simulink model "Microgrid_LCTLM_server"  (R2025b)
settings: Solver=ode3  StartTime=0.0  StopTime=1  FixedStep=params.sampleTime  RelTol=1e-3
InitFcn:
  | unitlmModelFile = get_param(bdroot, 'FileName');
  | if ~isempty(unitlmModelFile), addpath(fileparts(unitlmModelFile)); end
  | initialise_optimised_tlm_interface();
  | clear unitlmModelFile
StartFcn:
  | unitlmModelFile = get_param(bdroot, 'FileName'); if ~isempty(unitlmModelFile), addpath(fileparts(unitlmModelFile)); end; try, if exist('unitlm_timing_probe', 'file') == 2, unitlm_timing_probe('start', 'server', bdroot); else, warning('uniTLM:TimingProbeNotFound', 'unitlm_timing_probe.m not found on MATLAB path; timing probe disabled.'); end; catch unitlmTimingError, warning('uniTLM:TimingProbeFailed', 'unitlm_timing_probe failed: %s', unitlmTimingError.message); end; clear unitlmModelFile
StopFcn:
  | unitlmModelFile = get_param(bdroot, 'FileName'); if ~isempty(unitlmModelFile), addpath(fileparts(unitlmModelFile)); end; try, if exist('unitlm_timing_probe', 'file') == 2, unitlm_timing_probe('stop', 'server', bdroot); else, warning('uniTLM:TimingProbeNotFound', 'unitlm_timing_probe.m not found on MATLAB path; timing probe disabled.'); end; catch unitlmTimingError, warning('uniTLM:TimingProbeFailed', 'unitlm_timing_probe failed: %s', unitlmTimingError.message); end; clear unitlmModelFile
  | %% StopFcn: save TLM server-side results
  | 
  | modelName = bdroot;
  | modelFile = get_param(modelName, 'FileName');
  | 
  | if isempty(modelFile)
  |     modelDir = pwd;
  | else
  |     modelDir = fileparts(modelFile);
  | end
  | 
  | resultDir = fullfile(modelDir, 'result');
  | 
  | if ~exist(resultDir, 'dir')
  |     mkdir(resultDir);
  | end
  | 
  | % Server-side workspace variables
  | variableNames = {
  |     'server_voltage'
  |     'server_current'
  |     'server_PQ'
  | };
  | 
  | serverTLMData = struct();
  | 
  | for k = 1:numel(variableNames)
  | 
  |     originalName = variableNames{k};
  |     saveName = [originalName, '_TLM'];
  | 
  |     if evalin('base', sprintf('exist(''%s'', ''var'')', originalName))
  |         serverTLMData.(saveName) = evalin('base', originalName);
  |     else
  |         warning( ...
  |             'StopFcn:MissingVariable', ...
  |             'Variable "%s" was not found in the base workspace.', ...
  |             originalName);
  |     end
  | end
  | 
  | % Save to result/server_TLM.mat
  | saveFile = fullfile(resultDir, 'server_TLM.mat');
  | save(saveFile, '-struct', 'serverTLMData');
  | 
  | fprintf('TLM server-side results saved to:\n%s\n', saveFile);
values from neighbouring files (symbols this model uses):
  Cf = Cf_pu*Cb    [initialize_unitlm_microgrid.m]
  f = logspace(log10(fMin), log10(fMax), nFrequency).'    [fit_non_heaviside_line_rational.m]    (also in initialize_unitlm_microgrid.m = 50)
  fsw1 = 10e3    (= 10000)    [initialize_unitlm_microgrid.m]
  hr_lp_a = interface.hr_lp_a    [initialise_optimised_tlm_interface.m]
  hr_lp_b = interface.hr_lp_b    [initialise_optimised_tlm_interface.m]
  Ip = 2*P/(3*Vp)    [initialize_unitlm_microgrid.m]
  L1 = L1_pu*Lb    [initialize_unitlm_microgrid.m]
  L2 = L2_pu*Lb    [initialize_unitlm_microgrid.m]
  L3 = L3_pu*Lb    [initialize_unitlm_microgrid.m]
  L4 = L4_pu*Lb    [initialize_unitlm_microgrid.m]
  L_leakageinductance_1 = windingInductance(primaryWindingIndex)    [initialise_optimised_tlm_interface.m]
  L_magnetisation_1 = transformer.LmPu*primaryZbase/omegaNominal    [initialise_optimised_tlm_interface.m]
  L_remain_server = interface.L_remain_server    [initialise_optimised_tlm_interface.m]
  Lc = Lc_pu*Lb    [initialize_unitlm_microgrid.m]
  Lf2 = Lf2_pu*Lb    [initialize_unitlm_microgrid.m]
  line_aHr = interface.line_aHr    [initialise_optimised_tlm_interface.m]    (also in initialize_unitlm_microgrid.m = real(line_aHr))
  line_aZc = interface.line_aZc    [initialise_optimised_tlm_interface.m]    (also in initialize_unitlm_microgrid.m = real(line_aZc))
  line_bHr = interface.line_bHr    [initialise_optimised_tlm_interface.m]    (also in initialize_unitlm_microgrid.m = real(line_bHr))
  line_bZc = interface.line_bZc    [initialise_optimised_tlm_interface.m]    (also in initialize_unitlm_microgrid.m = real(line_bZc))
  P = 5e6    (= 5000000)    [initialize_unitlm_microgrid.m]
  params = varargin{1}    [Client_co.m]    (also in Client_co_TLM.m; Server_co.m; Server_co_TLM.m; initialise_optimised_tlm_interface.m = config.cosimParams)
  R1 = R1_pu*Zb    [initialize_unitlm_microgrid.m]
  R2 = R2_pu*Zb    [initialize_unitlm_microgrid.m]
  R3 = R3_pu*Zb    [initialize_unitlm_microgrid.m]
  R4 = R4_pu*Zb    [initialize_unitlm_microgrid.m]
  R_copperloss_1 = windingResistance(primaryWindingIndex)    [initialise_optimised_tlm_interface.m]
  R_coreloss_1 = transformer.RmPu*primaryZbase    [initialise_optimised_tlm_interface.m]
  R_remain_server = interface.R_remain_server    [initialise_optimised_tlm_interface.m]
  Rbreaker = Rbreaker_pu*Zb    [initialize_unitlm_microgrid.m]
  Rdamp = Rf    [initialize_unitlm_microgrid.m]
  Rf = Rf_pu*Zb    [initialize_unitlm_microgrid.m]
  Rload1 = Vp/Ip    [initialize_unitlm_microgrid.m]
  Rload2 = Vp/Ip    [initialize_unitlm_microgrid.m]
  Rload3 = Vp/Ip    [initialize_unitlm_microgrid.m]
  Rv_pu = 0.1    [initialize_unitlm_microgrid.m]
  Sxfmr = 6.3e6    (= 6300000)    [initialize_unitlm_microgrid.m]
  Vac = sqrt(2)*Vline/sqrt(3)    [initialize_unitlm_microgrid.m]
  Vhv = 66e3    (= 66000)    [initialize_unitlm_microgrid.m]
  Vline = 690    [initialize_unitlm_microgrid.m]
  Vp = Vac    [initialize_unitlm_microgrid.m]
  Wb = 2*pi*f    (= 314.159265359)    [initialize_unitlm_microgrid.m]
  Xv_pu = 0.3    [initialize_unitlm_microgrid.m]
  Zc_base_L = interface.Zc_base_L    [initialise_optimised_tlm_interface.m]
  Zc_base_R = interface.Zc_base_R    [initialise_optimised_tlm_interface.m]
undefined symbols (not defined in the file or in its folder): DiscIntNeverNeededParam, DPL, dspblkCoreblockFVToolHelper, gcbh, Lline1
libraries: spsThreePhaseSeriesRLCBranchLib x18, spsControlledVoltageSourceLib x12, spsThreePhaseVIMeasurementLib x7, spsabctodq0Lib x6, simulink x4, slpidlib x4, spsThreePhaseBreakerLib x4, SimplusGT x3, spsThreePhaseTransformerTwoWindingsLib x3, spsPower3phInstantaneousLib x2, spsdq0toabcLib x2, spsDistributedParametersLineLib x1
(part 2 of 4)

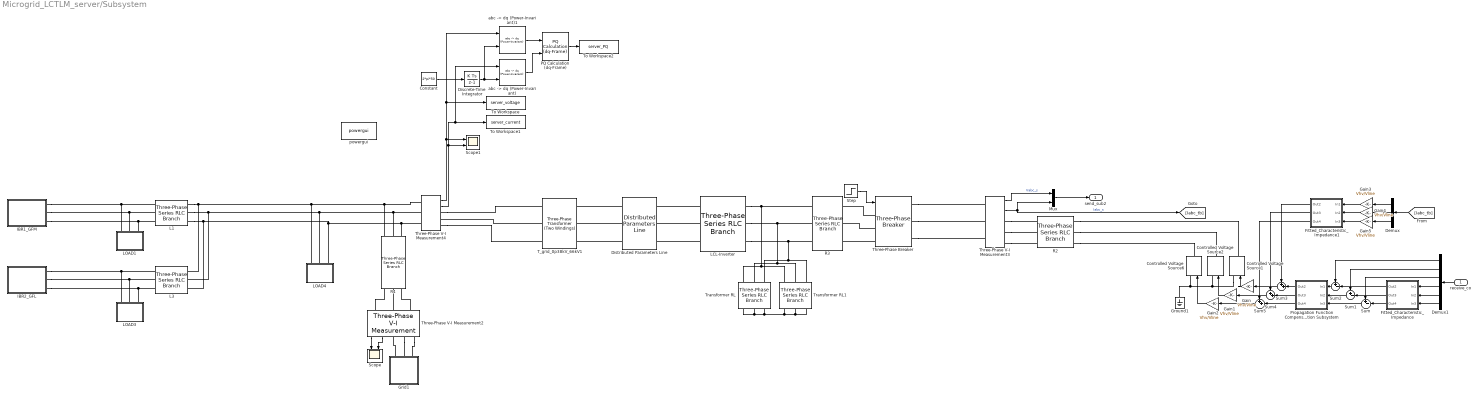
== system Microgrid_LCTLM_server/Subsystem ==
  receive_co : Inport
  Constant : Constant  Value=2*pi*50
  Controlled Voltage Source1 : spsControlledVoltageSourceLib/Controlled Voltage Source  Initialize=on  Source_Type=AC  Amplitude=0  Phase=0  Frequency=0  Measurements=None
  Controlled Voltage Source2 : spsControlledVoltageSourceLib/Controlled Voltage Source  Initialize=on  Source_Type=AC  Amplitude=0  Phase=0  Frequency=0  Measurements=None
  Controlled Voltage Source6 : spsControlledVoltageSourceLib/Controlled Voltage Source  Initialize=on  Source_Type=AC  Amplitude=0  Phase=0  Frequency=0  Measurements=None
  Demux : Demux  Outputs=3
  Demux1 : Demux  Outputs=6
  Discrete-Time Integrator : DiscreteIntegrator  SampleTime=-1  ICPrevOutput=DiscIntNeverNeededParam  ICPrevScaledInput=DiscIntNeverNeededParam
  Distributed Parameters Line : spsDistributedParametersLineLib/Distributed Parameters Line  Phases=3  Length=DPL.originalLength  Frequency=DPL.freq  Resistance=DPL.R  Inductance=DPL.L  Capacitance=DPL.C  x1=[-0.0002325 0 0 0;-0.000232 0 0 0;-0.0002315 0 0 0;-0.000231 0 0 0;-0.0002305 0 0 0;-0.00023 0 0 0;-0.0002295 0 0 0;-0.000229 0 0 0;-0.0002285 0 0 0;-0.000228 0 0 0;-0.0002275 0 0 0;-0.000227 0 0 0;-0.0002265 0 0 0;-0.000226 0 0 0;-0.0002255 0 0 0;-0.000225 0 0 0;-0.0002245 0 0 0;-0.000224 0 0 0;-0.0002235 0 0 0;-0.000223 0 0 0;-0.0002225 0 0 0;-0.000222 0 0 0;-0.0002215 0 0 0;-0.000221 0 0 0;-0.0002205 0 0 0;-0.00022 0 0 0;-0.0002195 0 0 0;-0.000219 0 0 0;-0.0002185 0 0 0;-0.000218 0 0 0;-0.0002175 0 0 0;-0.000217 0 0 0;-0.0002165 0 0 0;-0.000216 0 0 0;-0.0002155 0 0 0;-0.000215 0 0 0;-0.0002145 0 0 0;-0.000214 0 0 0;-0.0002135 0 0 0;-0.000213 0 0 0;-0.0002125 0 0 0;-0.000212 0 0 0;-0.0002115 0 0 0;-0.000211 0 0 0;-0.0002105 0 0 0;-0.00021 0 0 0;-0.0002095 0 0 0;-0.000209 0 0 0;-0.0002085 0 0 0;-0.000208 0 0 0;-0.0002075 0 0 0;-0.000207 0 0 0;-0.0002065 0 0 0;-0.000206 0 0 0;-0.0002055 0 0 0;-0.000205 0 0 0;-0.0002045 0 0 0;-0.000204 0 0 0;-0.0002035 0 0 0;-0.000203 0 0 0;-0.0002025 0 0 0;-0.000202 0 0 0;-0.0002015 0 0 0;-0.000201 0 0 0;-0.0002005 0 0 0;-0.0002 0 0 0;-0.0001995 0 0 0;-0.000199 0 0 0;-0.0001985 0 0 0;-0.000198 0 0 0;-0.0001975 0 0 0;-0.000197 0 0 0;-0.0001965 0 0 0;-0.000196 0 0 0;-0.0001955 0 0 0;-0.000195 0 0 0;-0.0001945 0 0 0;-0.000194 0 0 0;-0.0001935 0 0 0;-0.000193 0 0 0;-0.0001925 0 0 0;-0.000192 0 0 0;-0.0001915 0 0 0;-0.000191 0 0 0;-0.0001905 0 0 0;-0.00019 0 0 0;-0.0001895 0 0 0;-0.000189 0 0 0;-0.0001885 0 0 0;-0.000188 0 0 0;-0.0001875 0 0 0;-0.000187 0 0 0;-0.0001865 0 0 0;-0.000186 0 0 0;-0.0001855 0 0 0;-0.000185 0 0 0;-0.0001845 0 0 0;-0.000184 0 0 0;-0.0001835 0 0 0;-0.000183 0 0 0;-0.0001825 0 0 0;-0.000182 0 0 0;-0.0001815 0 0 0;-0.000181 0 0 0;-0.0001805 0 0 0;-0.00018 0 0 0;-0.0001795 0 0 0;-0.000179 0 0 0;-0.0001785 0 0 0;-0.000178 0 0 0;-0.0001775 0 0 0;-0.000177 0 0 0;-0.0001765 0 0 0;-0.000176 0 0 0;-0.0001755 0 0 0;-0.000175 0 0 0;-0.0001745 0 0 0;-0.000174 0 0 0;-0.0001735 0 0 0;-0.000173 0 0 0;-0.0001725 0 0 0;-0.000172 0 0 0;-0.0001715 0 0 0;-0.000171 0 0 0;-0.0001705 0 0 0;-0.00017 0 0 0;-0.0001695 0 0 0;-0.000169 0 0 0;-0.0001685 0 0 0;-0.000168 0 0 0;-0.0001675 0 0 0;-0.000167 0 0 0;-0.0001665 0 0 0;-0.000166 0 0 0;-0.0001655 0 0 0;-0.000165 0 0 0;-0.0001645 0 0 0;-0.000164 0 0 0;-0.0001635 0 0 0;-0.000163 0 0 0;-0.0001625 0 0 0;-0.000162 0 0 0;-0.0001615 0 0 0;-0.000161 0 0 0;-0.0001605 0 0 0;-0.00016 0 0 0;-0.0001595 0 0 0;-0.000159 0 0 0;-0.0001585 0 0 0;-0.000158 0 0 0;-0.0001575 0 0 0;-0.000157 0 0 0;-0.0001565 0 0 0;-0.000156 0 0 0;-0.0001555 0 0 0;-0.000155 0 0 0;-0.0001545 0 0 0;-0.000154 0 0 0;-0.0001535 0 0 0;-0.000153 0 0 0;-0.0001525 0 0 0;-0.000152 0 0 0;-0.0001515 0 0 0;-0.000151 0 0 0;-0.0001505 0 0 0;-0.00015 0 0 0;-0.0001495 0 0 0;-0.000149 0 0 0;-0.0001485 0 0 0;-0.000148 0 0 0;-0.0001475 0 0 0;-0.000147 0 0 0;-0.0001465 0 0 0;-0.000146 0 0 0;-0.0001455 0 0 0;-0.000145 0 0 0;-0.0001445 0 0 0;-0.000144 0 0 0;-0.0001435 0 0 0;-0.000143 0 0 0;-0.0001425 0 0 0;-0.000142 0 0 0;-0.0001415 0 0 0;-0.000141 0 0 0;-0.0001405 0 0 0;-0.00014 0 0 0;-0.0001395 0 0 0;-0.000139 0 0 0;-0.0001385 0 0 0;-0.000138 0 0 0;-0.0001375 0 0 0;-0.000137 0 0 0;-0.0001365 0 0 0;-0.000136 0 0 0;-0.0001355 0 0 0;-0.000135 0 0 0;-0.0001345 0 0 0;-0.000134 0 0 0;-0.0001335 0 0 0;-0.000133 0 0 0;-0.0001325 0 0 0;-0.000132 0 0 0;-0.0001315 0 0 0;-0.000131 0 0 0;-0.0001305 0 0 0;-0.00013 0 0 0;-0.0001295 0 0 0;-0.000129 0 0 0;-0.0001285 0 0 0;-0.000128 0 0 0;-0.0001275 0 0 0;-0.000127 0 0 0;-0.0001265 0 0 0;-0.000126 0 0 0;-0.0001255 0 0 0;-0.000125 0 0 0;-0.0001245 0 0 0;-0.000124 0 0 0;-0.0001235 0 0 0;-0.000123 0 0 0;-0.0001225 0 0 0;-0.000122 0 0 0;-0.0001215 0 0 0;-0.000121 0 0 0;-0.0001205 0 0 0;-0.00012 0 0 0;-0.0001195 0 0 0;-0.000119 0 0 0;-0.0001185 0 0 0;-0.000118 0 0 0;-0.0001175 0 0 0;-0.000117 0 0 0;-0.0001165 0 0 0;-0.000116 0 0 0;-0.0001155 0 0 0;-0.000115 0 0 0;-0.0001145 0 0 0;-0.000114 0 0 0;-0.0001135 0 0 0;-0.000113 0 0 0;-0.0001125 0 0 0;-0.000112 0 0 0;-0.0001115 0 0 0 ...(+3413 chars)]  x2=[-0.0002325 0 0 0;-0.000232 0 0 0;-0.0002315 0 0 0;-0.000231 0 0 0;-0.0002305 0 0 0;-0.00023 0 0 0;-0.0002295 0 0 0;-0.000229 0 0 0;-0.0002285 0 0 0;-0.000228 0 0 0;-0.0002275 0 0 0;-0.000227 0 0 0;-0.0002265 0 0 0;-0.000226 0 0 0;-0.0002255 0 0 0;-0.000225 0 0 0;-0.0002245 0 0 0;-0.000224 0 0 0;-0.0002235 0 0 0;-0.000223 0 0 0;-0.0002225 0 0 0;-0.000222 0 0 0;-0.0002215 0 0 0;-0.000221 0 0 0;-0.0002205 0 0 0;-0.00022 0 0 0;-0.0002195 0 0 0;-0.000219 0 0 0;-0.0002185 0 0 0;-0.000218 0 0 0;-0.0002175 0 0 0;-0.000217 0 0 0;-0.0002165 0 0 0;-0.000216 0 0 0;-0.0002155 0 0 0;-0.000215 0 0 0;-0.0002145 0 0 0;-0.000214 0 0 0;-0.0002135 0 0 0;-0.000213 0 0 0;-0.0002125 0 0 0;-0.000212 0 0 0;-0.0002115 0 0 0;-0.000211 0 0 0;-0.0002105 0 0 0;-0.00021 0 0 0;-0.0002095 0 0 0;-0.000209 0 0 0;-0.0002085 0 0 0;-0.000208 0 0 0;-0.0002075 0 0 0;-0.000207 0 0 0;-0.0002065 0 0 0;-0.000206 0 0 0;-0.0002055 0 0 0;-0.000205 0 0 0;-0.0002045 0 0 0;-0.000204 0 0 0;-0.0002035 0 0 0;-0.000203 0 0 0;-0.0002025 0 0 0;-0.000202 0 0 0;-0.0002015 0 0 0;-0.000201 0 0 0;-0.0002005 0 0 0;-0.0002 0 0 0;-0.0001995 0 0 0;-0.000199 0 0 0;-0.0001985 0 0 0;-0.000198 0 0 0;-0.0001975 0 0 0;-0.000197 0 0 0;-0.0001965 0 0 0;-0.000196 0 0 0;-0.0001955 0 0 0;-0.000195 0 0 0;-0.0001945 0 0 0;-0.000194 0 0 0;-0.0001935 0 0 0;-0.000193 0 0 0;-0.0001925 0 0 0;-0.000192 0 0 0;-0.0001915 0 0 0;-0.000191 0 0 0;-0.0001905 0 0 0;-0.00019 0 0 0;-0.0001895 0 0 0;-0.000189 0 0 0;-0.0001885 0 0 0;-0.000188 0 0 0;-0.0001875 0 0 0;-0.000187 0 0 0;-0.0001865 0 0 0;-0.000186 0 0 0;-0.0001855 0 0 0;-0.000185 0 0 0;-0.0001845 0 0 0;-0.000184 0 0 0;-0.0001835 0 0 0;-0.000183 0 0 0;-0.0001825 0 0 0;-0.000182 0 0 0;-0.0001815 0 0 0;-0.000181 0 0 0;-0.0001805 0 0 0;-0.00018 0 0 0;-0.0001795 0 0 0;-0.000179 0 0 0;-0.0001785 0 0 0;-0.000178 0 0 0;-0.0001775 0 0 0;-0.000177 0 0 0;-0.0001765 0 0 0;-0.000176 0 0 0;-0.0001755 0 0 0;-0.000175 0 0 0;-0.0001745 0 0 0;-0.000174 0 0 0;-0.0001735 0 0 0;-0.000173 0 0 0;-0.0001725 0 0 0;-0.000172 0 0 0;-0.0001715 0 0 0;-0.000171 0 0 0;-0.0001705 0 0 0;-0.00017 0 0 0;-0.0001695 0 0 0;-0.000169 0 0 0;-0.0001685 0 0 0;-0.000168 0 0 0;-0.0001675 0 0 0;-0.000167 0 0 0;-0.0001665 0 0 0;-0.000166 0 0 0;-0.0001655 0 0 0;-0.000165 0 0 0;-0.0001645 0 0 0;-0.000164 0 0 0;-0.0001635 0 0 0;-0.000163 0 0 0;-0.0001625 0 0 0;-0.000162 0 0 0;-0.0001615 0 0 0;-0.000161 0 0 0;-0.0001605 0 0 0;-0.00016 0 0 0;-0.0001595 0 0 0;-0.000159 0 0 0;-0.0001585 0 0 0;-0.000158 0 0 0;-0.0001575 0 0 0;-0.000157 0 0 0;-0.0001565 0 0 0;-0.000156 0 0 0;-0.0001555 0 0 0;-0.000155 0 0 0;-0.0001545 0 0 0;-0.000154 0 0 0;-0.0001535 0 0 0;-0.000153 0 0 0;-0.0001525 0 0 0;-0.000152 0 0 0;-0.0001515 0 0 0;-0.000151 0 0 0;-0.0001505 0 0 0;-0.00015 0 0 0;-0.0001495 0 0 0;-0.000149 0 0 0;-0.0001485 0 0 0;-0.000148 0 0 0;-0.0001475 0 0 0;-0.000147 0 0 0;-0.0001465 0 0 0;-0.000146 0 0 0;-0.0001455 0 0 0;-0.000145 0 0 0;-0.0001445 0 0 0;-0.000144 0 0 0;-0.0001435 0 0 0;-0.000143 0 0 0;-0.0001425 0 0 0;-0.000142 0 0 0;-0.0001415 0 0 0;-0.000141 0 0 0;-0.0001405 0 0 0;-0.00014 0 0 0;-0.0001395 0 0 0;-0.000139 0 0 0;-0.0001385 0 0 0;-0.000138 0 0 0;-0.0001375 0 0 0;-0.000137 0 0 0;-0.0001365 0 0 0;-0.000136 0 0 0;-0.0001355 0 0 0;-0.000135 0 0 0;-0.0001345 0 0 0;-0.000134 0 0 0;-0.0001335 0 0 0;-0.000133 0 0 0;-0.0001325 0 0 0;-0.000132 0 0 0;-0.0001315 0 0 0;-0.000131 0 0 0;-0.0001305 0 0 0;-0.00013 0 0 0;-0.0001295 0 0 0;-0.000129 0 0 0;-0.0001285 0 0 0;-0.000128 0 0 0;-0.0001275 0 0 0;-0.000127 0 0 0;-0.0001265 0 0 0;-0.000126 0 0 0;-0.0001255 0 0 0;-0.000125 0 0 0;-0.0001245 0 0 0;-0.000124 0 0 0;-0.0001235 0 0 0;-0.000123 0 0 0;-0.0001225 0 0 0;-0.000122 0 0 0;-0.0001215 0 0 0;-0.000121 0 0 0;-0.0001205 0 0 0;-0.00012 0 0 0;-0.0001195 0 0 0;-0.000119 0 0 0;-0.0001185 0 0 0;-0.000118 0 0 0;-0.0001175 0 0 0;-0.000117 0 0 0;-0.0001165 0 0 0;-0.000116 0 0 0;-0.0001155 0 0 0;-0.000115 0 0 0;-0.0001145 0 0 0;-0.000114 0 0 0;-0.0001135 0 0 0;-0.000113 0 0 0;-0.0001125 0 0 0;-0.000112 0 0 0;-0.0001115 0 0 0 ...(+3413 chars)]  x3=[-0.0002325 0 0 0;-0.000232 0 0 0;-0.0002315 0 0 0;-0.000231 0 0 0;-0.0002305 0 0 0;-0.00023 0 0 0;-0.0002295 0 0 0;-0.000229 0 0 0;-0.0002285 0 0 0;-0.000228 0 0 0;-0.0002275 0 0 0;-0.000227 0 0 0;-0.0002265 0 0 0;-0.000226 0 0 0;-0.0002255 0 0 0;-0.000225 0 0 0;-0.0002245 0 0 0;-0.000224 0 0 0;-0.0002235 0 0 0;-0.000223 0 0 0;-0.0002225 0 0 0;-0.000222 0 0 0;-0.0002215 0 0 0;-0.000221 0 0 0;-0.0002205 0 0 0;-0.00022 0 0 0;-0.0002195 0 0 0;-0.000219 0 0 0;-0.0002185 0 0 0;-0.000218 0 0 0;-0.0002175 0 0 0;-0.000217 0 0 0;-0.0002165 0 0 0;-0.000216 0 0 0;-0.0002155 0 0 0;-0.000215 0 0 0;-0.0002145 0 0 0;-0.000214 0 0 0;-0.0002135 0 0 0;-0.000213 0 0 0;-0.0002125 0 0 0;-0.000212 0 0 0;-0.0002115 0 0 0;-0.000211 0 0 0;-0.0002105 0 0 0;-0.00021 0 0 0;-0.0002095 0 0 0;-0.000209 0 0 0;-0.0002085 0 0 0;-0.000208 0 0 0;-0.0002075 0 0 0;-0.000207 0 0 0;-0.0002065 0 0 0;-0.000206 0 0 0;-0.0002055 0 0 0;-0.000205 0 0 0;-0.0002045 0 0 0;-0.000204 0 0 0;-0.0002035 0 0 0;-0.000203 0 0 0;-0.0002025 0 0 0;-0.000202 0 0 0;-0.0002015 0 0 0;-0.000201 0 0 0;-0.0002005 0 0 0;-0.0002 0 0 0;-0.0001995 0 0 0;-0.000199 0 0 0;-0.0001985 0 0 0;-0.000198 0 0 0;-0.0001975 0 0 0;-0.000197 0 0 0;-0.0001965 0 0 0;-0.000196 0 0 0;-0.0001955 0 0 0;-0.000195 0 0 0;-0.0001945 0 0 0;-0.000194 0 0 0;-0.0001935 0 0 0;-0.000193 0 0 0;-0.0001925 0 0 0;-0.000192 0 0 0;-0.0001915 0 0 0;-0.000191 0 0 0;-0.0001905 0 0 0;-0.00019 0 0 0;-0.0001895 0 0 0;-0.000189 0 0 0;-0.0001885 0 0 0;-0.000188 0 0 0;-0.0001875 0 0 0;-0.000187 0 0 0;-0.0001865 0 0 0;-0.000186 0 0 0;-0.0001855 0 0 0;-0.000185 0 0 0;-0.0001845 0 0 0;-0.000184 0 0 0;-0.0001835 0 0 0;-0.000183 0 0 0;-0.0001825 0 0 0;-0.000182 0 0 0;-0.0001815 0 0 0;-0.000181 0 0 0;-0.0001805 0 0 0;-0.00018 0 0 0;-0.0001795 0 0 0;-0.000179 0 0 0;-0.0001785 0 0 0;-0.000178 0 0 0;-0.0001775 0 0 0;-0.000177 0 0 0;-0.0001765 0 0 0;-0.000176 0 0 0;-0.0001755 0 0 0;-0.000175 0 0 0;-0.0001745 0 0 0;-0.000174 0 0 0;-0.0001735 0 0 0;-0.000173 0 0 0;-0.0001725 0 0 0;-0.000172 0 0 0;-0.0001715 0 0 0;-0.000171 0 0 0;-0.0001705 0 0 0;-0.00017 0 0 0;-0.0001695 0 0 0;-0.000169 0 0 0;-0.0001685 0 0 0;-0.000168 0 0 0;-0.0001675 0 0 0;-0.000167 0 0 0;-0.0001665 0 0 0;-0.000166 0 0 0;-0.0001655 0 0 0;-0.000165 0 0 0;-0.0001645 0 0 0;-0.000164 0 0 0;-0.0001635 0 0 0;-0.000163 0 0 0;-0.0001625 0 0 0;-0.000162 0 0 0;-0.0001615 0 0 0;-0.000161 0 0 0;-0.0001605 0 0 0;-0.00016 0 0 0;-0.0001595 0 0 0;-0.000159 0 0 0;-0.0001585 0 0 0;-0.000158 0 0 0;-0.0001575 0 0 0;-0.000157 0 0 0;-0.0001565 0 0 0;-0.000156 0 0 0;-0.0001555 0 0 0;-0.000155 0 0 0;-0.0001545 0 0 0;-0.000154 0 0 0;-0.0001535 0 0 0;-0.000153 0 0 0;-0.0001525 0 0 0;-0.000152 0 0 0;-0.0001515 0 0 0;-0.000151 0 0 0;-0.0001505 0 0 0;-0.00015 0 0 0;-0.0001495 0 0 0;-0.000149 0 0 0;-0.0001485 0 0 0;-0.000148 0 0 0;-0.0001475 0 0 0;-0.000147 0 0 0;-0.0001465 0 0 0;-0.000146 0 0 0;-0.0001455 0 0 0;-0.000145 0 0 0;-0.0001445 0 0 0;-0.000144 0 0 0;-0.0001435 0 0 0;-0.000143 0 0 0;-0.0001425 0 0 0;-0.000142 0 0 0;-0.0001415 0 0 0;-0.000141 0 0 0;-0.0001405 0 0 0;-0.00014 0 0 0;-0.0001395 0 0 0;-0.000139 0 0 0;-0.0001385 0 0 0;-0.000138 0 0 0;-0.0001375 0 0 0;-0.000137 0 0 0;-0.0001365 0 0 0;-0.000136 0 0 0;-0.0001355 0 0 0;-0.000135 0 0 0;-0.0001345 0 0 0;-0.000134 0 0 0;-0.0001335 0 0 0;-0.000133 0 0 0;-0.0001325 0 0 0;-0.000132 0 0 0;-0.0001315 0 0 0;-0.000131 0 0 0;-0.0001305 0 0 0;-0.00013 0 0 0;-0.0001295 0 0 0;-0.000129 0 0 0;-0.0001285 0 0 0;-0.000128 0 0 0;-0.0001275 0 0 0;-0.000127 0 0 0;-0.0001265 0 0 0;-0.000126 0 0 0;-0.0001255 0 0 0;-0.000125 0 0 0;-0.0001245 0 0 0;-0.000124 0 0 0;-0.0001235 0 0 0;-0.000123 0 0 0;-0.0001225 0 0 0;-0.000122 0 0 0;-0.0001215 0 0 0;-0.000121 0 0 0;-0.0001205 0 0 0;-0.00012 0 0 0;-0.0001195 0 0 0;-0.000119 0 0 0;-0.0001185 0 0 0;-0.000118 0 0 0;-0.0001175 0 0 0;-0.000117 0 0 0;-0.0001165 0 0 0;-0.000116 0 0 0;-0.0001155 0 0 0;-0.000115 0 0 0;-0.0001145 0 0 0;-0.000114 0 0 0;-0.0001135 0 0 0;-0.000113 0 0 0;-0.0001125 0 0 0;-0.000112 0 0 0;-0.0001115 0 0 0 ...(+3413 chars)]  x4=[-0.0002325 0 0 0;-0.000232 0 0 0;-0.0002315 0 0 0;-0.000231 0 0 0;-0.0002305 0 0 0;-0.00023 0 0 0;-0.0002295 0 0 0;-0.000229 0 0 0;-0.0002285 0 0 0;-0.000228 0 0 0;-0.0002275 0 0 0;-0.000227 0 0 0;-0.0002265 0 0 0;-0.000226 0 0 0;-0.0002255 0 0 0;-0.000225 0 0 0;-0.0002245 0 0 0;-0.000224 0 0 0;-0.0002235 0 0 0;-0.000223 0 0 0;-0.0002225 0 0 0;-0.000222 0 0 0;-0.0002215 0 0 0;-0.000221 0 0 0;-0.0002205 0 0 0;-0.00022 0 0 0;-0.0002195 0 0 0;-0.000219 0 0 0;-0.0002185 0 0 0;-0.000218 0 0 0;-0.0002175 0 0 0;-0.000217 0 0 0;-0.0002165 0 0 0;-0.000216 0 0 0;-0.0002155 0 0 0;-0.000215 0 0 0;-0.0002145 0 0 0;-0.000214 0 0 0;-0.0002135 0 0 0;-0.000213 0 0 0;-0.0002125 0 0 0;-0.000212 0 0 0;-0.0002115 0 0 0;-0.000211 0 0 0;-0.0002105 0 0 0;-0.00021 0 0 0;-0.0002095 0 0 0;-0.000209 0 0 0;-0.0002085 0 0 0;-0.000208 0 0 0;-0.0002075 0 0 0;-0.000207 0 0 0;-0.0002065 0 0 0;-0.000206 0 0 0;-0.0002055 0 0 0;-0.000205 0 0 0;-0.0002045 0 0 0;-0.000204 0 0 0;-0.0002035 0 0 0;-0.000203 0 0 0;-0.0002025 0 0 0;-0.000202 0 0 0;-0.0002015 0 0 0;-0.000201 0 0 0;-0.0002005 0 0 0;-0.0002 0 0 0;-0.0001995 0 0 0;-0.000199 0 0 0;-0.0001985 0 0 0;-0.000198 0 0 0;-0.0001975 0 0 0;-0.000197 0 0 0;-0.0001965 0 0 0;-0.000196 0 0 0;-0.0001955 0 0 0;-0.000195 0 0 0;-0.0001945 0 0 0;-0.000194 0 0 0;-0.0001935 0 0 0;-0.000193 0 0 0;-0.0001925 0 0 0;-0.000192 0 0 0;-0.0001915 0 0 0;-0.000191 0 0 0;-0.0001905 0 0 0;-0.00019 0 0 0;-0.0001895 0 0 0;-0.000189 0 0 0;-0.0001885 0 0 0;-0.000188 0 0 0;-0.0001875 0 0 0;-0.000187 0 0 0;-0.0001865 0 0 0;-0.000186 0 0 0;-0.0001855 0 0 0;-0.000185 0 0 0;-0.0001845 0 0 0;-0.000184 0 0 0;-0.0001835 0 0 0;-0.000183 0 0 0;-0.0001825 0 0 0;-0.000182 0 0 0;-0.0001815 0 0 0;-0.000181 0 0 0;-0.0001805 0 0 0;-0.00018 0 0 0;-0.0001795 0 0 0;-0.000179 0 0 0;-0.0001785 0 0 0;-0.000178 0 0 0;-0.0001775 0 0 0;-0.000177 0 0 0;-0.0001765 0 0 0;-0.000176 0 0 0;-0.0001755 0 0 0;-0.000175 0 0 0;-0.0001745 0 0 0;-0.000174 0 0 0;-0.0001735 0 0 0;-0.000173 0 0 0;-0.0001725 0 0 0;-0.000172 0 0 0;-0.0001715 0 0 0;-0.000171 0 0 0;-0.0001705 0 0 0;-0.00017 0 0 0;-0.0001695 0 0 0;-0.000169 0 0 0;-0.0001685 0 0 0;-0.000168 0 0 0;-0.0001675 0 0 0;-0.000167 0 0 0;-0.0001665 0 0 0;-0.000166 0 0 0;-0.0001655 0 0 0;-0.000165 0 0 0;-0.0001645 0 0 0;-0.000164 0 0 0;-0.0001635 0 0 0;-0.000163 0 0 0;-0.0001625 0 0 0;-0.000162 0 0 0;-0.0001615 0 0 0;-0.000161 0 0 0;-0.0001605 0 0 0;-0.00016 0 0 0;-0.0001595 0 0 0;-0.000159 0 0 0;-0.0001585 0 0 0;-0.000158 0 0 0;-0.0001575 0 0 0;-0.000157 0 0 0;-0.0001565 0 0 0;-0.000156 0 0 0;-0.0001555 0 0 0;-0.000155 0 0 0;-0.0001545 0 0 0;-0.000154 0 0 0;-0.0001535 0 0 0;-0.000153 0 0 0;-0.0001525 0 0 0;-0.000152 0 0 0;-0.0001515 0 0 0;-0.000151 0 0 0;-0.0001505 0 0 0;-0.00015 0 0 0;-0.0001495 0 0 0;-0.000149 0 0 0;-0.0001485 0 0 0;-0.000148 0 0 0;-0.0001475 0 0 0;-0.000147 0 0 0;-0.0001465 0 0 0;-0.000146 0 0 0;-0.0001455 0 0 0;-0.000145 0 0 0;-0.0001445 0 0 0;-0.000144 0 0 0;-0.0001435 0 0 0;-0.000143 0 0 0;-0.0001425 0 0 0;-0.000142 0 0 0;-0.0001415 0 0 0;-0.000141 0 0 0;-0.0001405 0 0 0;-0.00014 0 0 0;-0.0001395 0 0 0;-0.000139 0 0 0;-0.0001385 0 0 0;-0.000138 0 0 0;-0.0001375 0 0 0;-0.000137 0 0 0;-0.0001365 0 0 0;-0.000136 0 0 0;-0.0001355 0 0 0;-0.000135 0 0 0;-0.0001345 0 0 0;-0.000134 0 0 0;-0.0001335 0 0 0;-0.000133 0 0 0;-0.0001325 0 0 0;-0.000132 0 0 0;-0.0001315 0 0 0;-0.000131 0 0 0;-0.0001305 0 0 0;-0.00013 0 0 0;-0.0001295 0 0 0;-0.000129 0 0 0;-0.0001285 0 0 0;-0.000128 0 0 0;-0.0001275 0 0 0;-0.000127 0 0 0;-0.0001265 0 0 0;-0.000126 0 0 0;-0.0001255 0 0 0;-0.000125 0 0 0;-0.0001245 0 0 0;-0.000124 0 0 0;-0.0001235 0 0 0;-0.000123 0 0 0;-0.0001225 0 0 0;-0.000122 0 0 0;-0.0001215 0 0 0;-0.000121 0 0 0;-0.0001205 0 0 0;-0.00012 0 0 0;-0.0001195 0 0 0;-0.000119 0 0 0;-0.0001185 0 0 0;-0.000118 0 0 0;-0.0001175 0 0 0;-0.000117 0 0 0;-0.0001165 0 0 0;-0.000116 0 0 0;-0.0001155 0 0 0;-0.000115 0 0 0;-0.0001145 0 0 0;-0.000114 0 0 0;-0.0001135 0 0 0;-0.000113 0 0 0;-0.0001125 0 0 0;-0.000112 0 0 0;-0.0001115 0 0 0 ...(+3413 chars)]  x5=0.000232379000772445  V1=ones(3,3)  V2=ones(3,3)  I1=ones(3,3)  I2=ones(3,3)  nHarmo=1  Measurements=None  Decoupling=off  VsMag0=0  VrMag0=0  VsAngle0=0  VrAngle0=0  IsMag0=0  IrMag0=0  IsAngle0=0  IrAngle0=0
      settings: LibrarySourceBlock=sps_lib/Power Grid Elements/Distributed Parameters Line
  Fitted_Characteristic_Impedance : Subsystem
  Fitted_Characteristic_Impedance1 : Subsystem
  Gain{,1..5} (6 alike) : Gain  Gain=Vhv/Vline
  Grid1 : Subsystem
  Ground1 : spsGroundLib/Ground  LConnTagsString=a
  IBR1_GFM : Subsystem
  IBR2_GFL : Subsystem
  L1 : spsThreePhaseSeriesRLCBranchLib/Three-Phase Series RLC Branch  LConnTagsString=A|B|C  RConnTagsString=A|B|C  BranchType=RL  Resistance=R1  Inductance=L1  Capacitance=1e-6  Measurements=None
  L3 : spsThreePhaseSeriesRLCBranchLib/Three-Phase Series RLC Branch  LConnTagsString=A|B|C  RConnTagsString=A|B|C  BranchType=RL  Resistance=R3  Inductance=L3  Capacitance=1e-6  Measurements=None
  LCL-Inverter : spsThreePhaseSeriesRLCBranchLib/Three-Phase Series RLC Branch  LConnTagsString=A|B|C  RConnTagsString=A|B|C  BranchType=RL  Resistance=R_copperloss_1  Inductance=L_leakageinductance_1  Capacitance=1e-6  Measurements=None
  LOAD1 : Subsystem
  LOAD3 : Subsystem
  LOAD4 : Subsystem
  Mux : Mux  Inputs=2
  PQ Calculation (dq-Frame) : SimplusGT/PQ Calculation (dq-Frame)  SystemSampleTime=-1  VariantActivationTime=update diagram  EmptyChoice=off  PassThrough=off  PassThroughVariantControl=(default)  EmptyChoiceVariantControl=(default)  AllowFlexibleInterface=on  Latency=0  AutoFrameSizeCalculation=off
      settings: SourceProductName=Simplus Grid Tool
  Propagation Function Compensation Subsystem : Subsystem
  R2 : spsThreePhaseSeriesRLCBranchLib/Three-Phase Series RLC Branch  LConnTagsString=A|B|C  RConnTagsString=A|B|C  BranchType=RL  Resistance=Zc_base_R*(Vhv/Vline)^2  Inductance=Zc_base_L*(Vhv/Vline)^2  Capacitance=1e-6  Measurements=None
  R3 : spsThreePhaseSeriesRLCBranchLib/Three-Phase Series RLC Branch  LConnTagsString=A|B|C  RConnTagsString=A|B|C  BranchType=RL  Resistance=R_remain_server*(Vhv/Vline)^2  Inductance=L_remain_server*(Vhv/Vline)^2  Capacitance=1e-6  Measurements=None
  R4 : spsThreePhaseSeriesRLCBranchLib/Three-Phase Series RLC Branch  LConnTagsString=A|B|C  RConnTagsString=A|B|C  BranchType=RL  Resistance=R4  Inductance=L4  Capacitance=1e-6  Measurements=None
  Scope : Scope  NumInputPorts=2
      settings: ActiveDisplayYMinimum=-671.75144212722125  ActiveDisplayYMaximum=671.75144212722125
  Scope1 : Scope  NumInputPorts=2
      settings: ActiveDisplayYMinimum=-1278.7291215477867  ActiveDisplayYMaximum=1279.3125875681185  DataLoggingVariableName=ScopeData2
  Step : Step  Time=0.1  SampleTime=0
  Sum : Sum  Inputs=+-|
  Sum1 : Sum  Inputs=+-|
  Sum2 : Sum  Inputs=+-|
  Sum3 : Sum  Inputs=++|
  Sum4 : Sum  Inputs=++|
  Sum5 : Sum  Inputs=++|
  T_grid_0p38kV_66kV1 : spsThreePhaseTransformerTwoWindingsLib/Three-Phase Transformer (Two Windings)  Winding1Connection=Yg  Winding2Connection=Yg  CoreType=Three single-phase transformers  SetSaturation=off  Hysteresis=off  DataFile='hysteresis'  SetInitialFlux=off  Measurements=None  UNITS=pu  NominalPower=[Sxfmr, f]  Winding1=[Vhv, 0.002, 0.04]  Winding2=[Vline, 0.002, 0.04]  Rm=500  Lm=500  L0=0.5  Saturation=[ 0,0 ; 0.0024,1.2 ; 1.0,1.52 ]  InitialFluxes=[ 0.8 , -0.8 , 0.7 ]  BreakLoop=off  DiscreteSolver=Trapezoidal iterative  DataType=off  TransfoNumber=1
  Three-Phase V-I Measurement2 : spsThreePhaseVIMeasurementLib/Three-Phase V-I Measurement  VoltageMeasurement=phase-to-phase  SetLabelV=off  LabelV=Vabc1  Vpu=off  VpuLL=off  CurrentMeasurement=yes  SetLabelI=off  LabelI=Iabc3  Ipu=off  Pbase=100e6  Vbase=500e3  OutputType=Complex  PhasorSimulation=off  PSBequivalent=0
  Three-Phase V-I Measurement3 : spsThreePhaseVIMeasurementLib/Three-Phase V-I Measurement  VoltageMeasurement=phase-to-ground  SetLabelV=off  LabelV=Vabc_s  Vpu=off  VpuLL=off  CurrentMeasurement=yes  SetLabelI=off  LabelI=Iabc_s  Ipu=off  Pbase=100e6  Vbase=500e3  OutputType=Complex  PhasorSimulation=off  PSBequivalent=0
  Three-Phase V-I Measurement4 : spsThreePhaseVIMeasurementLib/Three-Phase V-I Measurement  VoltageMeasurement=phase-to-phase  SetLabelV=off  LabelV=Vabc1  Vpu=off  VpuLL=off  CurrentMeasurement=yes  SetLabelI=off  LabelI=Iabc3  Ipu=off  Pbase=100e6  Vbase=500e3  OutputType=Complex  PhasorSimulation=off  PSBequivalent=0
  Three-Phase Breaker : spsThreePhaseBreakerLib/Three-Phase Breaker  InitialState=open  SwitchA=on  SwitchB=on  SwitchC=on  SwitchTimes="[1/60  5/60]"  External=on  BreakerResistance=Rbreaker*(Vhv/Vline)^2  SnubberResistance=1e6*(Vhv/Vline)^2  SnubberCapacitance=inf  Measurements=None
  To Workspace : ToWorkspace  VariableName=server_voltage  SaveFormat=Timeseries  SampleTime=-1
  To Workspace1 : ToWorkspace  VariableName=server_current  SaveFormat=Timeseries  SampleTime=-1
  To Workspace2 : ToWorkspace  VariableName=server_PQ  SaveFormat=Timeseries  SampleTime=-1
  Transformer RL : spsThreePhaseSeriesRLCBranchLib/Three-Phase Series RLC Branch  LConnTagsString=A|B|C  RConnTagsString=A|B|C  BranchType=R  Resistance=R_coreloss_1  Inductance=L_magnetisation_1  Capacitance=1e-6  Measurements=None
  Transformer RL1 : spsThreePhaseSeriesRLCBranchLib/Three-Phase Series RLC Branch  LConnTagsString=A|B|C  RConnTagsString=A|B|C  BranchType=L  Resistance=R_coreloss_1  Inductance=L_magnetisation_1  Capacitance=1e-6  Measurements=None
  "abc -> dq (Power-Invariant)" : SimplusGT/abc -> dq (Power-Invariant)  SystemSampleTime=-1  VariantActivationTime=update diagram  EmptyChoice=off  PassThrough=off  PassThroughVariantControl=(default)  EmptyChoiceVariantControl=(default)  AllowFlexibleInterface=on  Latency=0  AutoFrameSizeCalculation=off
      settings: SourceProductName=Simplus Grid Tool
  "abc -> dq (Power-Invariant)1" : SimplusGT/abc -> dq (Power-Invariant)  SystemSampleTime=-1  VariantActivationTime=update diagram  EmptyChoice=off  PassThrough=off  PassThroughVariantControl=(default)  EmptyChoiceVariantControl=(default)  AllowFlexibleInterface=on  Latency=0  AutoFrameSizeCalculation=off
      settings: SourceProductName=Simplus Grid Tool
  powergui : spspowerguiLib/powergui  Priority=1  SimulationMode=Discrete  SampleTime=params.sampleTime  frequency=60  Iterations=50  frequencyindice=0  Pbase=100e6  ErrMax=1e-4  UnitsV=kV  UnitsW=MW  buscounter=0  FunctionMessages=off  echomessages=off  EnableUseOfTLC=off  CurrentSourceSwitches=off  DisableSnubberDevices=off  DisableRonSwitches=off  DisableVfSwitches=off  DisplayEquations=off  AutomaticDiscreteSolvers=off  SolverType=Tustin/Backward Euler (TBE)  Interpol=off  ExternalGateDelay=off  methode=off  Ts=100  x0status=blocks  SPID=on  SwTol=0  HookPort=off  NonlinearTolerance=1e-4  nMaxIteration=100  ContinueOnMaxIteration=off  RestoreLinks=warning  ResistiveCurrentMeasurement=off  Frange=[0:2:500]  Ylog=off  Xlog=on  ShowGrid=off  save=off  variable=ZData  structure=0  ZoomFFT=off  StartTime=0.0  cycles=1  DisplayStyle=1  fundamental=60  FreqAxis=off  MaxFrequency=1000  frequencyindicesteady=1  RmsSteady=1  display=off
  send_sub2 : Outport
  wires:
  Three-Phase V-I Measurement2/2 -> Scope/2
  Three-Phase V-I Measurement2/1 -> Scope/1
  Three-Phase V-I Measurement3/2 -> [Iabc_tb], Mux/2  "Iabc_s"
  Mux/1 -> send_sub2/1
  Three-Phase V-I Measurement3/1 -> Mux/1  "Vabc_s"
  Three-Phase V-I Measurement4/1 -> Scope1/1, "abc -> dq (Power-Invariant)1"/1, To Workspace/1
  Three-Phase V-I Measurement4/2 -> Scope1/2, "abc -> dq (Power-Invariant)"/1, To Workspace1/1
  Discrete-Time Integrator/1 -> "abc -> dq (Power-Invariant)1"/2, "abc -> dq (Power-Invariant)"/2
  Constant/1 -> Discrete-Time Integrator/1
  "abc -> dq (Power-Invariant)1"/1 -> PQ Calculation (dq-Frame)/1
  "abc -> dq (Power-Invariant)"/1 -> PQ Calculation (dq-Frame)/2
  PQ Calculation (dq-Frame)/1 -> To Workspace2/1
  Demux1/6 -> Fitted_Characteristic_Impedance/3(In3)
  Fitted_Characteristic_Impedance/3(Out4) -> Sum/2
  Fitted_Characteristic_Impedance/2(Out3) -> Sum1/2
  Demux1/5 -> Fitted_Characteristic_Impedance/2(In2)
  Demux1/3 -> Sum/1
  Sum2/1 -> Propagation Function Compensation Subsystem/1(In1)
  Sum/1 -> Propagation Function Compensation Subsystem/3(In3)
  Sum1/1 -> Propagation Function Compensation Subsystem/2(In2)
  Demux1/1 -> Sum2/1
  Demux1/2 -> Sum1/1
  Demux1/4 -> Fitted_Characteristic_Impedance/1(In1)
  Fitted_Characteristic_Impedance/1(Out2) -> Sum2/2
  receive_co/1 -> Demux1/1
  [Iabc_tb] -> Demux/1
  Gain/1 -> Controlled Voltage Source1/1
  Gain1/1 -> Controlled Voltage Source2/1
  Gain2/1 -> Controlled Voltage Source6/1
  Sum3/1 -> Gain/1
  Propagation Function Compensation Subsystem/1(Out2) -> Sum3/2
  Propagation Function Compensation Subsystem/2(Out3) -> Sum4/2
  Sum4/1 -> Gain1/1
  Sum5/1 -> Gain2/1
  Propagation Function Compensation Subsystem/3(Out4) -> Sum5/2
  Fitted_Characteristic_Impedance1/3(Out4) -> Sum5/1
  Fitted_Characteristic_Impedance1/2(Out3) -> Sum4/1
  Fitted_Characteristic_Impedance1/1(Out2) -> Sum3/1
  Demux/1 -> Gain3/1
  Gain3/1 -> Fitted_Characteristic_Impedance1/1(In1)
  Demux/2 -> Gain4/1
  Gain4/1 -> Fitted_Characteristic_Impedance1/2(In2)
  Demux/3 -> Gain5/1
  Gain5/1 -> Fitted_Characteristic_Impedance1/3(In3)
  Step/1 -> Three-Phase Breaker/1
  connections:
  IBR1_GFM/RConn2 -- L1/LConn2 -- LOAD1/LConn2
  LCL-Inverter/LConn1 -- R3/RConn1 -- Transformer RL/LConn1 -- Transformer RL1/LConn1
  Grid1/LConn1 -- Three-Phase V-I Measurement2/RConn1
  LOAD4/LConn1 -- Three-Phase V-I Measurement4/LConn1 -- R4/LConn1 -- L1/RConn1 -- L3/RConn1
  Three-Phase V-I Measurement2/LConn3 -- R4/RConn3
  L1/LConn1 -- IBR1_GFM/RConn1 -- LOAD1/LConn1
  L1/RConn2 -- Three-Phase V-I Measurement4/LConn2 -- R4/LConn2 -- LOAD4/LConn2 -- L3/RConn2
  Three-Phase V-I Measurement2/RConn2 -- Grid1/LConn2
  IBR1_GFM/RConn3 -- L1/LConn3 -- LOAD1/LConn3
  L1/RConn3 -- L3/RConn3 -- LOAD4/LConn3 -- Three-Phase V-I Measurement4/LConn3 -- R4/LConn3
  LOAD3/LConn1 -- IBR2_GFL/RConn1 -- L3/LConn1
  IBR2_GFL/RConn2 -- LOAD3/LConn2 -- L3/LConn2
  Three-Phase V-I Measurement2/RConn3 -- Grid1/LConn3
  Three-Phase V-I Measurement2/LConn1 -- R4/RConn1
  IBR2_GFL/RConn3 -- LOAD3/LConn3 -- L3/LConn3
  Three-Phase V-I Measurement2/LConn2 -- R4/RConn2
  Ground1/LConn1 -- Controlled Voltage Source1/LConn1 -- Controlled Voltage Source2/LConn1 -- Controlled Voltage Source6/LConn1
  Transformer RL/LConn2 -- LCL-Inverter/LConn2 -- R3/RConn2 -- Transformer RL1/LConn2
  Transformer RL/LConn3 -- LCL-Inverter/LConn3 -- R3/RConn3 -- Transformer RL1/LConn3
  Three-Phase V-I Measurement4/RConn1 -- T_grid_0p38kV_66kV1/RConn1
  T_grid_0p38kV_66kV1/RConn2 -- Three-Phase V-I Measurement4/RConn2
  Three-Phase V-I Measurement4/RConn3 -- T_grid_0p38kV_66kV1/RConn3
  Distributed Parameters Line/RConn1 -- T_grid_0p38kV_66kV1/LConn1
  Distributed Parameters Line/RConn2 -- T_grid_0p38kV_66kV1/LConn2
  Distributed Parameters Line/RConn3 -- T_grid_0p38kV_66kV1/LConn3
  Transformer RL/RConn1 -- Transformer RL/RConn2 -- Transformer RL1/RConn3 -- Transformer RL1/RConn2 -- Transformer RL1/RConn1 -- Transformer RL/RConn3
  LCL-Inverter/RConn1 -- Distributed Parameters Line/LConn1
  LCL-Inverter/RConn2 -- Distributed Parameters Line/LConn2
  LCL-Inverter/RConn3 -- Distributed Parameters Line/LConn3
  Three-Phase V-I Measurement3/RConn2 -- R2/RConn2
  Three-Phase V-I Measurement3/RConn3 -- R2/RConn3
  Three-Phase V-I Measurement3/RConn1 -- R2/RConn1
  R2/LConn1 -- Controlled Voltage Source1/RConn1
  R2/LConn2 -- Controlled Voltage Source2/RConn1
  R2/LConn3 -- Controlled Voltage Source6/RConn1
  Three-Phase Breaker/LConn3 -- R3/LConn3
  Three-Phase Breaker/LConn2 -- R3/LConn2
  Three-Phase Breaker/LConn1 -- R3/LConn1
  Three-Phase Breaker/RConn1 -- Three-Phase V-I Measurement3/LConn1
  Three-Phase Breaker/RConn2 -- Three-Phase V-I Measurement3/LConn2
  Three-Phase Breaker/RConn3 -- Three-Phase V-I Measurement3/LConn3
